simulink library "vmc"  (R2021b)
settings: Solver=VariableStepAuto  StartTime=0.0  StopTime=10.0  RelTol=1e-3
undefined symbols (not defined in the file): AVMC_ACCDeltaTqGradeGn_X_deg, AVMC_ACCDeltaTqIGain4OVRD_X_kph, AVMC_ACCDeltaTqIGain4OVRD_Y_mps2, AVMC_ACCDeltaTqIGain_X_kph, AVMC_ACCDeltaTqIGain_Y_mps2, AVMC_ACCDeltaTqPGain_X_kph, AVMC_ACCDeltaTqPGain_Y_kph, AVMC_ACCGradeofst_X_G, AVMC_ACCGradeofst_Y_pct, AVMC_ACCLoSpdTqLoLim4JP_X_kph, AVMC_ACCLoSpdTqLoLim4JP_Y_deg, AVMC_ACCLoSpdTqLowerLim_X_kph, AVMC_ACCLoSpdTqLowerLim_Y_deg, AVMC_ACCReqAccelGain_X_mps2, AVMC_ACCReqAccelGain_Y_enum, AVMC_ADSPosGFBDeltaTq_X_kph, AVMC_ADSPosGFBDeltaTq_Y_mps2, AVMC_AggressJerkPCT4AT_X_kph, AVMC_AggressJerkPCT_X_kph, AVMC_AggressLimitPCT4AT_X_kph, AVMC_AggressLimitPCT_X_kph, AVMC_DECGradeofst_X_G, AVMC_DECGradeofst_Y_pct, AVMC_DISCDeltaTqIGain_X_kph, AVMC_DISCDeltaTqIGain_Y_mps2, AVMC_DISCDeltaTqPGain_X_kph, AVMC_DISCDeltaTqPGain_Y_kph, AVMC_EPSForceSelect_X_enum, AVMC_EPSForceSelect_Y_enum, AVMC_EPSForceSelectD21_X_enum, AVMC_EPSForceSelectD21_Y_enum, AVMC_ESCRegenOut_X_kph, AVMC_ESCRegenOut_Y_Deg, AVMC_ESCRegenOutEnSpd_X_Deg, AVMC_EstPitchSlopeTs_X_kph, AVMC_GradeCompFlt_X_kph, AVMC_GyroYBandLo_X_Gps, AVMC_HoldResTq_X_kph, AVMC_ISOAccLimit_X_mps, AVMC_ISODecLimit_X_mps, AVMC_ISOJerk_X_mps, AVMC_LatESCRegenOut_X_kph, AVMC_LatESCRegenOut_Y_Deg, AVMC_LongAccDeadZone_X_kph, AVMC_LongAccFiltTsforP2_X_Gps, AVMC_MCPresBaseTq_X_bar, AVMC_MSAPedalOvrd_X_kph, AVMC_MSASpdBand_X_kph, AVMC_MSATqDownEndTq_X_kph, AVMC_MSATqDownTime_X_kph, AVMC_NegZCHoldTq_X_kph, AVMC_OPDDisSlideRate_X_Deg, AVMC_OVRD2ActSR2FCMCMD_X_mps2, AVMC_PedalTqRWhlRatio_X_Nm, AVMC_PedalTqRWhlRatio_Y_gps, AVMC_PedalTqRWhlSlipGain_X_rat, AVMC_PedalTqRWhlSlipGain_Y_kph, AVMC_PedalTqRWhSTRGGain_X_deg, AVMC_PedalTqRWhSTRGGain_Y_kph, AVMC_PosZCHoldTq_X_kph ... (+593)
libraries: hcu_lib x143, simulink x96, tqr x4, $bdroot x1, simulink_extras x1
(part 3 of 17)

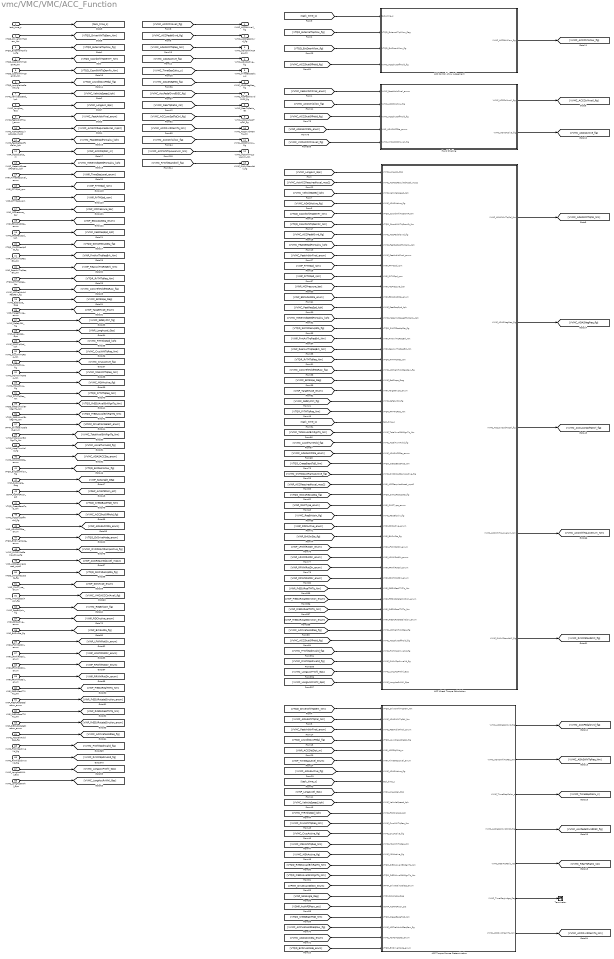
== system vmc/VMC/VMC/ACC_Function ==
  task_time_s : Inport
  VTQD_DriverWhlTqDem_Nm : Inport  Port=2
  VTQD_ExternalTqAllow_flg : Inport  Port=3
  VTQD_CoordWhlTqDemFr_Nm : Inport  Port=4
  VTQD_CoordWhlTqDemRr_Nm : Inport  Port=5
  VTQD_LowIdleAccPedal_flg : Inport  Port=6
  VVMC_VehicleSpeed_kph : Inport  Port=7
  VVMC_LongAcc_Gps : Inport  Port=8
  VVMC_FeatArbitrFinal_enum : Inport  Port=9
  VVMC_ActACCRequiredAccel_mps2 : Inport  Port=10
  VVMC_FeatSetSpdForCalcu_kph : Inport  Port=11
  VINP_ACCObjDist_m : Inport  Port=12
  VVMC_MeterIndSpeedForCalcu_kph : Inport  Port=13
  VINP_TimeGapLevel_enum : Inport  Port=14
  VINP_FrTMSpd_rpm : Inport  Port=15
  VINP_RrTMSpd_rpm : Inport  Port=16
  VINP_MCPressure_bar : Inport  Port=17
  VINP_ESCADASSta_enum : Inport  Port=18
  VVMC_FeatReqSpd_kph : Inport  Port=19
  VTQD_SWC2ResUpSta_flg : Inport  Port=20
  VINP_FrntAxlTrqReqBrk_Nm : Inport  Port=21
  VINP_RearAxlTrqReqBrk_Nm : Inport  Port=22
  VTQR_RrTMTqReq_Nm : Inport  Port=23
  VVMC_ACCVehHoldReqRaw_flg : Inport  Port=24
  VVMC_EstSlope_Deg : Inport  Port=25
  VINP_TargetType_enum : Inport  Port=26
  VVMC_SafetyCtrl_flg : Inport  Port=27
  VINP_LongAccel_Gps : Inport  Port=28
  VVMC_FrRrSlipSpd_kph : Inport  Port=29
  VVMC_CruzWhlTqReq_Nm : Inport  Port=30
  VVMC_CruzActive_flg : Inport  Port=31
  VVMC_MSAWhlTqReq_Nm : Inport  Port=32
  VVMC_MSAActive_flg : Inport  Port=33
  VTQR_FrTMTqReq_Nm : Inport  Port=34
  VTQD_RrEDUAvailBrkRgnTq_Nm : Inport  Port=35
  VTQD_FrEDUAvailBrkRgnTq_Nm : Inport  Port=36
  VPMM_DrivetrainSelect_enum : Inport  Port=37
  VVMC_TotalAvailBrkRgnTq_Nm : Inport  Port=38
  VVMC_AccelTurnHold_flg : Inport  Port=39
  VVMC_ADASACCSta_enum : Inport  Port=40
  VTQD_ExtDoorAllow_flg : Inport  Port=41
  VINP_SASAngle_Deg : Inport  Port=42
  VDHP_ActAPSPosn_pct : Inport  Port=43
  VTQD_CreepBaseTqD_Nm : Inport  Port=44
  VVMC_ACCShutOffHold_flg : Inport  Port=45
  VINP_ADASACCSta_enum : Inport  Port=46
  VTQD_EVDriveMode_enum : Inport  Port=47
  VVMC_OVRD2ActRampActive_flg : Inport  Port=48
  VINP_ACCRequiredAccel_mps2 : Inport  Port=49
  VTQD_SWC1ResUpSta_flg : Inport  Port=50
  VINP_SWCType_enum : Inport  Port=51
  VVMC_VMCACCCtrlAvail_flg : Inport  Port=52
  VVMC_ReqBrkJoin_flg : Inport  Port=53
  VINP_RDCActive_enum : Inport  Port=54
  VINP_BrkSwSta_flg : Inport  Port=55
  VINP_LFWhlRotDir_enum : Inport  Port=56
  VINP_LRWhlRotDir_enum : Inport  Port=57
  VINP_RFWhlRotDir_enum : Inport  Port=58
  VINP_RRWhlRotDir_enum : Inport  Port=59
  VINP_FrEDURealTMTq_Nm : Inport  Port=60
  VINP_FrEDURotateDirction_enum : Inport  Port=61
  VINP_RrEDURealTMTq_Nm : Inport  Port=62
  VINP_RrEDURotateDirction_enum : Inport  Port=63
  VVMC_ACCVehHoldReq_flg : Inport  Port=64
  VVMC_FrWhlSpdInvalid_flg : Inport  Port=65
  VVMC_RrWhlSpdInvalid_flg : Inport  Port=66
  VVMC_LongAccFrWhl_Gps : Inport  Port=67
  VVMC_LongAccRrWhl_Gps : Inport  Port=68
  ACC Control Allow Judgement : Subsystem
  ACC Torque Source Determination : Subsystem
  ACC Wheel Torque Calculation : Subsystem
  Hand Shaking : Subsystem
  Terminator : Terminator
  VVMC_ACCCtrlAvail_flg : Outport
  VVMC_ACCPedalOvrd_flg : Outport  Port=2
  VVMC_ADASWhlTqReq_Nm : Outport  Port=3
  VVMC_ADASActive_flg : Outport  Port=4
  VVMC_TimeGapCalcu_s : Outport  Port=5
  VVMC_ADASNegReq_flg : Outport  Port=6
  VVMC_AccPedalOvrdDISC_flg : Outport  Port=7
  VVMC_RearTqRatio_rat : Outport  Port=8
  VVMC_ACCLowSpdTqCtrl_flg : Outport  Port=9
  VVMC_ACCOvrdMemTq_Nm : Outport  Port=10
  VVMC_ACCCtrlAllow_flg : Outport  Port=11
  VVMC_ACCWhlTqLowerLim_Nm : Outport  Port=12
  VVMC_RrWhlStandstill_flg : Outport  Port=13
  wires:
  [VVMC_ACCCtrlAllow_flg] -> VVMC_ACCCtrlAllow_flg/1
  VVMC_VMCACCCtrlAvail_flg/1 -> [VVMC_VMCACCCtrlAvail_flg]
  [VVMC_VMCACCCtrlAvail_flg] -> Hand Shaking/5(VVMC_VMCACCCtrlAvail_flg)
  [VINP_SWCType_enum] -> ACC Wheel Torque Calculation/33(VINP_SWCType_enum)
  VINP_SWCType_enum/1 -> [VINP_SWCType_enum]
  [VTQD_SWC1ResUpSta_flg] -> ACC Wheel Torque Calculation/32(VTQD_SWC1ResUpSta_flg)
  VTQD_SWC1ResUpSta_flg/1 -> [VTQD_SWC1ResUpSta_flg]
  [VINP_ACCRequiredAccel_mps2] -> ACC Wheel Torque Calculation/31(VINP_ACCRequiredAccel_mps2)
  VINP_ACCRequiredAccel_mps2/1 -> [VINP_ACCRequiredAccel_mps2]
  [VVMC_OVRD2ActRampActive_flg] -> ACC Wheel Torque Calculation/30(VVMC_OVRD2ActRampActive_flg)
  VVMC_OVRD2ActRampActive_flg/1 -> [VVMC_OVRD2ActRampActive_flg]
  [VTQD_EVDriveMode_enum] -> ACC Torque Source Determination/24(VTQD_EVDriveMode_enum)
  VTQD_EVDriveMode_enum/1 -> [VTQD_EVDriveMode_enum]
  [VINP_ADASACCSta_enum] -> Hand Shaking/4(VINP_ADASACCSta_enum)
  VINP_ADASACCSta_enum/1 -> [VINP_ADASACCSta_enum]
  [VVMC_ACCShutOffHold_flg] -> Hand Shaking/3(VVMC_ACCShutOffHold_flg)
  VVMC_ACCShutOffHold_flg/1 -> [VVMC_ACCShutOffHold_flg]
  [VTQD_CreepBaseTqD_Nm] -> ACC Wheel Torque Calculation/29(VTQD_CreepBaseTqD_Nm)
  [VVMC_ADASACCSta_enum] -> ACC Torque Source Determination/23(VVMC_ADASACCSta_enum)
  [VVMC_ACCVehHoldReqRaw_flg] -> ACC Torque Source Determination/22(VVMC_ACCVehHoldReqRaw_flg)
  ACC Torque Source Determination/7(VVMC_ACCOvrdMemTq_Nm) -> [VVMC_ACCOvrdMemTq_Nm]
  [VVMC_ACCOvrdMemTq_Nm] -> VVMC_ACCOvrdMemTq_Nm/1
  [VTQD_CreepBaseTqD_Nm] -> ACC Torque Source Determination/21(VTQD_CreepBaseTqD_Nm)
  VTQD_CreepBaseTqD_Nm/1 -> [VTQD_CreepBaseTqD_Nm]
  VDHP_ActAPSPosn_pct/1 -> [VDHP_ActAPSPosn_pct]
  [VDHP_ActAPSPosn_pct] -> ACC Torque Source Determination/20(VDHP_ActAPSPosn_pct)
  VINP_SASAngle_Deg/1 -> [VINP_SASAngle_Deg]
  [VINP_SASAngle_Deg] -> ACC Torque Source Determination/19(VINP_SASAngle_Deg)
  VTQD_ExtDoorAllow_flg/1 -> [VTQD_ExtDoorAllow_flg]
  [VTQD_ExtDoorAllow_flg] -> ACC Control Allow Judgement/3(VTQD_ExtDoorAllow_flg)
  ACC Torque Source Determination/6(VVMC_TimeGapJudge_flag) -> Terminator/1
  [VVMC_ADASACCSta_enum] -> ACC Wheel Torque Calculation/28(VVMC_ADASACCSta_enum)
  VVMC_ADASACCSta_enum/1 -> [VVMC_ADASACCSta_enum]
  [VVMC_AccelTurnHold_flg] -> ACC Wheel Torque Calculation/27(VVMC_AccelTurnHold_flg)
  VVMC_AccelTurnHold_flg/1 -> [VVMC_AccelTurnHold_flg]
  [VVMC_TotalAvailBrkRgnTq_Nm] -> ACC Wheel Torque Calculation/26(VVMC_TotalAvailBrkRgnTq_Nm)
  VVMC_TotalAvailBrkRgnTq_Nm/1 -> [VVMC_TotalAvailBrkRgnTq_Nm]
  [task_time_s] -> ACC Wheel Torque Calculation/25(task_time_s)
  [VPMM_DrivetrainSelect_enum] -> ACC Torque Source Determination/18(VPMM_DrivetrainSelect_enum)
  VPMM_DrivetrainSelect_enum/1 -> [VPMM_DrivetrainSelect_enum]
  [VVMC_ACCLowSpdTqCtrl_flg] -> VVMC_ACCLowSpdTqCtrl_flg/1
  ACC Wheel Torque Calculation/3(VVMC_ACCLowSpdTqCtrl_flg) -> [VVMC_ACCLowSpdTqCtrl_flg]
  [VTQD_FrEDUAvailBrkRgnTq_Nm] -> ACC Torque Source Determination/17(VTQD_FrEDUAvailBrkRgnTq_Nm)
  [VTQD_RrEDUAvailBrkRgnTq_Nm] -> ACC Torque Source Determination/16(VTQD_RrEDUAvailBrkRgnTq_Nm)
  VTQD_FrEDUAvailBrkRgnTq_Nm/1 -> [VTQD_FrEDUAvailBrkRgnTq_Nm]
  VTQD_RrEDUAvailBrkRgnTq_Nm/1 -> [VTQD_RrEDUAvailBrkRgnTq_Nm]
  VTQR_FrTMTqReq_Nm/1 -> [VTQR_FrTMTqReq_Nm]
  [VTQR_FrTMTqReq_Nm] -> ACC Wheel Torque Calculation/24(VTQR_FrTMTqReq_Nm)
  [VVMC_MSAActive_flg] -> ACC Torque Source Determination/15(VVMC_MSAActive_flg)
  [VVMC_MSAWhlTqReq_Nm] -> ACC Torque Source Determination/14(VVMC_MSAWhlTqReq_Nm)
  [VVMC_CruzActive_flg] -> ACC Torque Source Determination/13(VVMC_CruzActive_flg)
  [VVMC_CruzWhlTqReq_Nm] -> ACC Torque Source Determination/12(VVMC_CruzWhlTqReq_Nm)
  VVMC_CruzWhlTqReq_Nm/1 -> [VVMC_CruzWhlTqReq_Nm]
  VVMC_CruzActive_flg/1 -> [VVMC_CruzActive_flg]
  VVMC_MSAWhlTqReq_Nm/1 -> [VVMC_MSAWhlTqReq_Nm]
  VVMC_MSAActive_flg/1 -> [VVMC_MSAActive_flg]
  [VVMC_FrRrSlipSpd_kph] -> ACC Torque Source Determination/11(VVMC_FrRrSlipSpd_kph)
  [VVMC_VehicleSpeed_kph] -> ACC Torque Source Determination/10(VVMC_VehicleSpeed_kph)
  VVMC_FrRrSlipSpd_kph/1 -> [VVMC_FrRrSlipSpd_kph]
  VINP_LongAccel_Gps/1 -> [VINP_LongAccel_Gps]
  [VVMC_RearTqRatio_rat] -> VVMC_RearTqRatio_rat/1
  ACC Torque Source Determination/5(VVMC_RearTqRatio_rat) -> [VVMC_RearTqRatio_rat]
  [VINP_LongAccel_Gps] -> ACC Torque Source Determination/9(VINP_LongAccel_Gps)
  [VVMC_SafetyCtrl_flg] -> ACC Wheel Torque Calculation/23(VVMC_SafetyCtrl_flg)
  VVMC_SafetyCtrl_flg/1 -> [VVMC_SafetyCtrl_flg]
  [task_time_s] -> ACC Torque Source Determination/8(task_time_s)
  VINP_TargetType_enum/1 -> [VINP_TargetType_enum]
  [VINP_TargetType_enum] -> ACC Wheel Torque Calculation/22(VINP_TargetType_enum)
  [VVMC_EstSlope_Deg] -> ACC Wheel Torque Calculation/21(VVMC_EstSlope_Deg)
  VVMC_EstSlope_Deg/1 -> [VVMC_EstSlope_Deg]
  [VVMC_ACCVehHoldReqRaw_flg] -> ACC Wheel Torque Calculation/20(VVMC_ACCVehHoldReqRaw_flg)
  VVMC_ACCVehHoldReqRaw_flg/1 -> [VVMC_ACCVehHoldReqRaw_flg]
  [VVMC_AccPedalOvrdDISC_flg] -> VVMC_AccPedalOvrdDISC_flg/1
  ACC Torque Source Determination/4(VVMC_AccPedalOvrdDISC_flg) -> [VVMC_AccPedalOvrdDISC_flg]
  [VTQR_RrTMTqReq_Nm] -> ACC Wheel Torque Calculation/19(VTQR_RrTMTqReq_Nm)
  VTQR_RrTMTqReq_Nm/1 -> [VTQR_RrTMTqReq_Nm]
  [VVMC_ADASNegReq_flg] -> VVMC_ADASNegReq_flg/1
  ACC Wheel Torque Calculation/2(VVMC_ADASNegReq_flg) -> [VVMC_ADASNegReq_flg]
  [VINP_RearAxlTrqReqBrk_Nm] -> ACC Wheel Torque Calculation/18(VINP_RearAxlTrqReqBrk_Nm)
  [VINP_FrntAxlTrqReqBrk_Nm] -> ACC Wheel Torque Calculation/17(VINP_FrntAxlTrqReqBrk_Nm)
  [VTQD_SWC2ResUpSta_flg] -> ACC Wheel Torque Calculation/16(VTQD_SWC2ResUpSta_flg)
  [VVMC_MeterIndSpeedForCalcu_kph] -> ACC Wheel Torque Calculation/15(VVMC_MeterIndSpeedForCalcu_kph)
  VINP_RearAxlTrqReqBrk_Nm/1 -> [VINP_RearAxlTrqReqBrk_Nm]
  VINP_FrntAxlTrqReqBrk_Nm/1 -> [VINP_FrntAxlTrqReqBrk_Nm]
  VTQD_SWC2ResUpSta_flg/1 -> [VTQD_SWC2ResUpSta_flg]
  [VVMC_FeatSetSpdForCalcu_kph] -> ACC Wheel Torque Calculation/8(VVMC_FeatSetSpdForCalcu_kph)
  VVMC_FeatSetSpdForCalcu_kph/1 -> [VVMC_FeatSetSpdForCalcu_kph]
  [VTQD_LowIdleAccPedal_flg] -> ACC Torque Source Determination/4(VTQD_LowIdleAccPedal_flg)
  VTQD_LowIdleAccPedal_flg/1 -> [VTQD_LowIdleAccPedal_flg]
  [VVMC_FeatArbitrFinal_enum] -> ACC Torque Source Determination/3(VVMC_FeatArbitrFinal_enum)
  [VVMC_ACCPedalOvrd_flg] -> ACC Wheel Torque Calculation/7(VVMC_ACCPedalOvrd_flg)
  VTQD_CoordWhlTqDemFr_Nm/1 -> [VTQD_CoordWhlTqDemFr_Nm]
  VTQD_CoordWhlTqDemRr_Nm/1 -> [VTQD_CoordWhlTqDemRr_Nm]
  [VTQD_CoordWhlTqDemRr_Nm] -> ACC Wheel Torque Calculation/6(VTQD_CoordWhlTqDemRr_Nm)
  [VTQD_CoordWhlTqDemFr_Nm] -> ACC Wheel Torque Calculation/5(VTQD_CoordWhlTqDemFr_Nm)
  [VVMC_ADASWhlTqReq_Nm] -> VVMC_ADASWhlTqReq_Nm/1
  ACC Torque Source Determination/2(VVMC_ADASWhlTqReq_Nm) -> [VVMC_ADASWhlTqReq_Nm]
  [VVMC_ADASActive_flg] -> VVMC_ADASActive_flg/1
  [VVMC_ACCCtrlAllow_flg] -> Hand Shaking/2(VVMC_ACCCtrlAllow_flg)
  task_time_s/1 -> [task_time_s]
  [VVMC_ADASActive_flg] -> ACC Wheel Torque Calculation/4(VVMC_ADASActive_flg)
  Hand Shaking/2(VVMC_ADASActive_flg) -> [VVMC_ADASActive_flg]
  [VVMC_FeatArbitrFinal_enum] -> Hand Shaking/1(VVMC_FeatArbitrFinal_enum)
  ACC Torque Source Determination/1(VVMC_ACCPedalOvrd_flg) -> [VVMC_ACCPedalOvrd_flg]
  [VVMC_ADASWhlTqCal_Nm] -> ACC Torque Source Determination/2(VVMC_ADASWhlTqCal_Nm)
  [VTQD_DriverWhlTqDem_Nm] -> ACC Torque Source Determination/1(VTQD_DriverWhlTqDem_Nm)
  ACC Wheel Torque Calculation/1(VVMC_ADASWhlTqCal_Nm) -> [VVMC_ADASWhlTqCal_Nm]
  [VVMC_VehicleSpeed_kph] -> ACC Wheel Torque Calculation/3(VVMC_VehicleSpeed_kph)
  [VVMC_ActACCRequiredAccel_mps2] -> ACC Wheel Torque Calculation/2(VVMC_ActACCRequiredAccel_mps2)
  [VVMC_LongAcc_Gps] -> ACC Wheel Torque Calculation/1(VVMC_LongAcc_Gps)
  VTQD_DriverWhlTqDem_Nm/1 -> [VTQD_DriverWhlTqDem_Nm]
  VVMC_VehicleSpeed_kph/1 -> [VVMC_VehicleSpeed_kph]
  VTQD_ExternalTqAllow_flg/1 -> [VTQD_ExternalTqAllow_flg]
  [VVMC_ACCCtrlAvail_flg] -> VVMC_ACCCtrlAvail_flg/1
  VVMC_ActACCRequiredAccel_mps2/1 -> [VVMC_ActACCRequiredAccel_mps2]
  VVMC_FeatArbitrFinal_enum/1 -> [VVMC_FeatArbitrFinal_enum]
  VVMC_LongAcc_Gps/1 -> [VVMC_LongAcc_Gps]
  Hand Shaking/1(VVMC_ACCCtrlAvail_flg) -> [VVMC_ACCCtrlAvail_flg]
  [VVMC_ACCPedalOvrd_flg] -> VVMC_ACCPedalOvrd_flg/1
  VVMC_MeterIndSpeedForCalcu_kph/1 -> [VVMC_MeterIndSpeedForCalcu_kph]
  VINP_ACCObjDist_m/1 -> [VINP_ACCObjDist_m]
  VINP_TimeGapLevel_enum/1 -> [VINP_TimeGapLevel_enum]
  [VINP_ACCObjDist_m] -> ACC Torque Source Determination/5(VINP_ACCObjDist_m)
  [VINP_TimeGapLevel_enum] -> ACC Torque Source Determination/6(VINP_TimeGapLevel_enum)
  ACC Torque Source Determination/3(VVMC_TimeGapCalcu_s) -> [VVMC_TimeGapCalcu_s]
  [VVMC_TimeGapCalcu_s] -> VVMC_TimeGapCalcu_s/1
  [task_time_s] -> ACC Control Allow Judgement/1(task_time_s)
  ACC Control Allow Judgement/1(VVMC_ACCCtrlAllow_flg) -> [VVMC_ACCCtrlAllow_flg]
  [VTQD_ExternalTqAllow_flg] -> ACC Control Allow Judgement/2(VTQD_ExternalTqAllow_flag)
  [VVMC_FeatArbitrFinal_enum] -> ACC Wheel Torque Calculation/9(VVMC_FeatArbitrFinal_enum)
  VINP_ESCADASSta_enum/1 -> [VINP_ESCADASSta_enum]
  VINP_MCPressure_bar/1 -> [VINP_MCPressure_bar]
  VINP_RrTMSpd_rpm/1 -> [VINP_RrTMSpd_rpm]
  VINP_FrTMSpd_rpm/1 -> [VINP_FrTMSpd_rpm]
  [VINP_FrTMSpd_rpm] -> ACC Wheel Torque Calculation/10(VINP_FrTMSpd_rpm)
  [VINP_RrTMSpd_rpm] -> ACC Wheel Torque Calculation/11(VINP_RrTMSpd_rpm)
  [VINP_MCPressure_bar] -> ACC Wheel Torque Calculation/12(VINP_MCPressure_bar)
  [VINP_ESCADASSta_enum] -> ACC Wheel Torque Calculation/13(VINP_ESCADASSta_enum)
  [VVMC_ADASActive_flg] -> ACC Torque Source Determination/7(VVMC_ADASActive_flg)
  VVMC_FeatReqSpd_kph/1 -> [VVMC_FeatReqSpd_kph]
  [VVMC_FeatReqSpd_kph] -> ACC Wheel Torque Calculation/14(VVMC_FeatReqSpd_kph)
  VVMC_ReqBrkJoin_flg/1 -> [VVMC_ReqBrkJoin_flg]
  [VVMC_ReqBrkJoin_flg] -> ACC Wheel Torque Calculation/34(VVMC_ReqBrkJoin_flg)
  [VVMC_ACCWhlTqLowerLim_Nm] -> VVMC_ACCWhlTqLowerLim_Nm/1
  ACC Wheel Torque Calculation/4(VVMC_ACCWhlTqLowerLim_Nm) -> [VVMC_ACCWhlTqLowerLim_Nm]
  VINP_RDCActive_enum/1 -> [VINP_RDCActive_enum]
  [VINP_RDCActive_enum] -> ACC Wheel Torque Calculation/35(VINP_RDCActive_enum)
  VINP_BrkSwSta_flg/1 -> [VINP_BrkSwSta_flg]
  [VINP_BrkSwSta_flg] -> ACC Wheel Torque Calculation/36(VINP_BrkSwSta_flg)
  VINP_LFWhlRotDir_enum/1 -> [VINP_LFWhlRotDir_enum]
  VINP_RFWhlRotDir_enum/1 -> [VINP_RFWhlRotDir_enum]
  VINP_LRWhlRotDir_enum/1 -> [VINP_LRWhlRotDir_enum]
  VINP_RRWhlRotDir_enum/1 -> [VINP_RRWhlRotDir_enum]
  [VINP_LFWhlRotDir_enum] -> ACC Wheel Torque Calculation/37(VINP_LFWhlRotDir_enum)
  [VINP_LRWhlRotDir_enum] -> ACC Wheel Torque Calculation/38(VINP_LRWhlRotDir_enum)
  [VINP_RFWhlRotDir_enum] -> ACC Wheel Torque Calculation/39(VINP_RFWhlRotDir_enum)
  [VINP_RRWhlRotDir_enum] -> ACC Wheel Torque Calculation/40(VINP_RRWhlRotDir_enum)
  VINP_FrEDURotateDirction_enum/1 -> [VINP_FrEDURotateDirction_enum]
  VINP_RrEDURotateDirction_enum/1 -> [VINP_RrEDURotateDirction_enum]
  VINP_FrEDURealTMTq_Nm/1 -> [VINP_FrEDURealTMTq_Nm]
  VINP_RrEDURealTMTq_Nm/1 -> [VINP_RrEDURealTMTq_Nm]
  [VINP_FrEDURealTMTq_Nm] -> ACC Wheel Torque Calculation/41(VINP_FrEDURealTMTq_Nm)
  [VINP_FrEDURotateDirction_enum] -> ACC Wheel Torque Calculation/42(VINP_FrEDURotateDirction_enum)
  [VINP_RrEDURealTMTq_Nm] -> ACC Wheel Torque Calculation/43(VINP_RrEDURealTMTq_Nm)
  [VINP_RrEDURotateDirction_enum] -> ACC Wheel Torque Calculation/44(VINP_RrEDURotateDirction_enum)
  [VVMC_RrWhlStandstill_flg] -> VVMC_RrWhlStandstill_flg/1
  ACC Wheel Torque Calculation/5(VVMC_RrWhlStandstill_flg) -> [VVMC_RrWhlStandstill_flg]
  [VVMC_ACCShutOffHold_flg] -> ACC Control Allow Judgement/4(VVMC_ACCShutOffHold_flg)
  VVMC_ACCVehHoldReq_flg/1 -> [VVMC_ACCVehHoldReq_flg]
  [VVMC_ACCVehHoldReq_flg] -> ACC Wheel Torque Calculation/45(VVMC_ACCVehHoldReq_flg)
  [VVMC_ACCShutOffHold_flg] -> ACC Wheel Torque Calculation/46(VVMC_ACCShutOffHold_flg)
  VVMC_FrWhlSpdInvalid_flg/1 -> [VVMC_FrWhlSpdInvalid_flg]
  VVMC_RrWhlSpdInvalid_flg/1 -> [VVMC_RrWhlSpdInvalid_flg]
  VVMC_LongAccFrWhl_Gps/1 -> [VVMC_LongAccFrWhl_Gps]
  VVMC_LongAccRrWhl_Gps/1 -> [VVMC_LongAccRrWhl_Gps]
  [VVMC_FrWhlSpdInvalid_flg] -> ACC Wheel Torque Calculation/47(VVMC_FrWhlSpdInvalid_flg)
  [VVMC_RrWhlSpdInvalid_flg] -> ACC Wheel Torque Calculation/48(VVMC_RrWhlSpdInvalid_flg)
  [VVMC_LongAccFrWhl_Gps] -> ACC Wheel Torque Calculation/49(VVMC_LongAccFrWhl_Gps)
  [VVMC_LongAccRrWhl_Gps] -> ACC Wheel Torque Calculation/50(VVMC_LongAccRrWhl_Gps)

== system vmc/VMC/VMC/APS function ==
  VTQD_ExternalTqAllow_flg : Inport
  VTQD_ExtShiftAllow_flg : Inport  Port=2
  VTQD_ExtDoorAllow_flg : Inport  Port=3
  VTQD_GearActualPosn_enum : Inport  Port=4
  VINP_APSVMCReqA_flg : Inport  Port=5
  VINP_APSShiftPosnReq_enum : Inport  Port=6
  VINP_APSSpeedCMD_kph : Inport  Port=7
  task_time_s : Inport  Port=8
  VINP_SCPSystemMode_enum : Inport  Port=9
  VVMC_ADASActive_flg : Inport  Port=10
  VTQD_APSStaSys_enum : Inport  Port=11
  VTQD_APSDecReqA_flg : Inport  Port=12
  VTQD_APSDecReq_mps2 : Inport  Port=13
  VTQD_APSReq_enum : Inport  Port=14
  VINP_APSStaSystem_enum : Inport  Port=15
  VINP_APSDecReqA_flg : Inport  Port=16
  VINP_APSDecReq_mps2 : Inport  Port=17
  VINP_APSReq_enum : Inport  Port=18
  VVMC_VehicleSpeed_kph : Inport  Port=19
  VVMC_CruzActive_flg : Inport  Port=20
  VINP_CAASVMCReqA_flg : Inport  Port=21
  VINP_ADASACCSta_enum : Inport  Port=22
  VINP_BrkSwSta_flg : Inport  Port=23
  VINP_MCPressure_bar : Inport  Port=24
  VINP_BrkPedalPos_pct : Inport  Port=25
  VINP_ACCObjDist_m : Inport  Port=26
  VVMC_MeterIndSpeedForCalcu_kph : Inport  Port=27
  VDDM_VCURAPSErrLv2_flg : Inport  Port=28
  VDDM_VCURAPSErrLv3_flg : Inport  Port=29
  VTQD_EPBCarWashMode_flg : Inport  Port=30
  CAAS HandShake : Subsystem
  Command Determination1 : Subsystem
  Hand Shake : Subsystem
  Signal Rounting : Subsystem
  Subsystem : Subsystem
  VVMC_APSCtrlAvail_flg : Outport
  VVMC_APSActive_flg : Outport  Port=2
  VVMC_CAASCtrlAvail_flg : Outport  Port=3
  VVMC_CAASActive_flg : Outport  Port=4
  VVMC_APSSpeedCMD_kph : Outport  Port=5
  VVMC_APSShiftPosnReq_enum : Outport  Port=6
  VVMC_APSStaSys_enum : Outport  Port=7
  VVMC_APSDecReqA_flg : Outport  Port=8
  VVMC_APSDecReq_mps2 : Outport  Port=9
  VVMC_APSReq_enum : Outport  Port=10
  VVMC_SetACCDisableAPS_flg : Outport  Port=11
  wires:
  VDDM_VCURAPSErrLv2_flg/1 -> [VDDM_VCURAPSErrLv2_flg]
  VTQD_EPBCarWashMode_flg/1 -> [VTQD_EPBCarWashMode_flg]
  VDDM_VCURAPSErrLv3_flg/1 -> [VDDM_VCURAPSErrLv3_flg]
  [VTQD_EPBCarWashMode_flg] -> Hand Shake/10(VTQD_EPBCarWashMode_flg)
  [VTQD_GearActualPosn_enum] -> Hand Shake/7(VTQD_GearActualPosn_enum)
  [VDDM_VCURAPSErrLv2_flg] -> Hand Shake/8(VDDM_VCURAPSErrLv2_flg)
  [VDDM_VCURAPSErrLv3_flg] -> Hand Shake/9(VDDM_VCURAPSErrLv3_flg)
  [VVMC_VehicleSpeed_kph] -> Subsystem/8(VVMC_VehicleSpeed_kph)
  [VVMC_SetACCDisableAPS_flg] -> Signal Rounting/14(VVMC_SetACCDisableAPS_flg)
  VVMC_MeterIndSpeedForCalcu_kph/1 -> [VVMC_MeterIndSpeedForCalcu_kph]
  VINP_ACCObjDist_m/1 -> [VINP_ACCObjDist_m]
  VINP_BrkPedalPos_pct/1 -> [VINP_BrkPedalPos_pct]
  VINP_MCPressure_bar/1 -> [VINP_MCPressure_bar]
  VINP_BrkSwSta_flg/1 -> [VINP_BrkSwSta_flg]
  VINP_ADASACCSta_enum/1 -> [VINP_ADASACCSta_enum]
  Subsystem/1(VVMC_SetACCDisableAPS_flg) -> [VVMC_SetACCDisableAPS_flg], VVMC_SetACCDisableAPS_flg/1
  [VINP_ADASACCSta_enum] -> Subsystem/1(VINP_ADASACCSta_enum)
  [VVMC_MeterIndSpeedForCalcu_kph] -> Subsystem/7(VVMC_MeterIndSpeedForCalcu_kph)
  [VINP_ACCObjDist_m] -> Subsystem/6(VINP_ACCObjDist_m)
  [VINP_BrkSwSta_flg] -> Subsystem/3(VINP_BrkSwSta_flg)
  [VINP_MCPressure_bar] -> Subsystem/2(VINP_MCPressure_bar)
  [VINP_BrkPedalPos_pct] -> Subsystem/4(VINP_BrkPedalPos_pct)
  [VTQD_APSDecReqA_flg] -> Subsystem/5(VTQD_APSDecReqA_flg)
  VINP_CAASVMCReqA_flg/1 -> [VINP_CAASVMCReqA_flg]
  VVMC_CruzActive_flg/1 -> [VVMC_CruzActive_flg]
  VVMC_VehicleSpeed_kph/1 -> [VVMC_VehicleSpeed_kph]
  [VTQD_APSReq_enum] -> Signal Rounting/9(VTQD_APSReq_enum)
  [VINP_APSReq_enum] -> Signal Rounting/13(VINP_APSReq_enum)
  [VINP_APSDecReq_mps2] -> Signal Rounting/12(VINP_APSDecReq_mps2)
  [VINP_APSDecReqA_flg] -> Signal Rounting/11(VINP_APSDecReqA_flg)
  [VTQD_APSDecReq_mps2] -> Signal Rounting/8(VTQD_APSDecReq_mps2)
  [VTQD_APSDecReqA_flg] -> Signal Rounting/7(VTQD_APSDecReqA_flg)
  [VINP_APSStaSystem_enum] -> Signal Rounting/10(VINP_APSStaSystem_enum)
  [VTQD_APSStaSys_enum] -> Signal Rounting/6(VTQD_APSStaSys_enum)
  VINP_APSDecReqA_flg/1 -> [VINP_APSDecReqA_flg]
  VINP_APSStaSystem_enum/1 -> [VINP_APSStaSystem_enum]
  VINP_APSReq_enum/1 -> [VINP_APSReq_enum]
  VINP_APSDecReq_mps2/1 -> [VINP_APSDecReq_mps2]
  Signal Rounting/4(VVMC_APSReq_enum) -> VVMC_APSReq_enum/1
  [VINP_APSSpeedCMD_kph] -> Command Determination1/4(VINP_APSSpeedCMD_kph)
  Command Determination1/2(VVMC_APSShiftPosnReq_enum) -> VVMC_APSShiftPosnReq_enum/1
  [VINP_APSShiftPosnReq_enum] -> Command Determination1/3(VINP_APSShiftPosnReq_enum)
  [VINP_APSStaSystem_enum] -> Command Determination1/2(VINP_APSStaSys_enum)
  [VTQD_GearActualPosn_enum] -> Signal Rounting/4(VTQD_GearActualPosn_enum)
  [VINP_SCPSystemMode_enum] -> Signal Rounting/1(VINP_SCPSystemMode_enum)
  [VVMC_APSActive_flg] -> Signal Rounting/2(VVMC_APSActive_flg)
  Signal Rounting/1(VVMC_APSStaSys_enum) -> VVMC_APSStaSys_enum/1
  [VVMC_ADASActive_flg] -> Signal Rounting/3(VVMC_ADASActive_flg)
  Signal Rounting/3(VVMC_APSDecReq_mps2) -> VVMC_APSDecReq_mps2/1
  Signal Rounting/2(VVMC_APSDecReqA_flg) -> VVMC_APSDecReqA_flg/1
  [VVMC_APSActive_flg] -> Command Determination1/1(VVMC_APSActive_flg)
  [VVMC_CAASActive_flg] -> Signal Rounting/5(VVMC_CAASActive_flg)
  Command Determination1/1(VVMC_APSSpeedCMD_kph) -> VVMC_APSSpeedCMD_kph/1
  [VTQD_ExternalTqAllow_flg] -> Hand Shake/2(VTQD_ExternalTqAllow_flg)
  [task_time_s] -> Hand Shake/1(task_time_s)
  [VTQD_ExtShiftAllow_flg] -> Hand Shake/3(VTQD_ExtShiftAllow_flg)
  [VINP_APSStaSystem_enum] -> Hand Shake/5(VINP_APSStaSys_enum)
  CAAS HandShake/2(VVMC_CAASActive_flg) -> [VVMC_CAASActive_flg], VVMC_CAASActive_flg/1
  [VINP_CAASVMCReqA_flg] -> CAAS HandShake/5(VINP_CAASVMCReqA_flg)
  [task_time_s] -> CAAS HandShake/4(task_time_s)
  CAAS HandShake/1(VVMC_CAASCtrlAvail_flg) -> VVMC_CAASCtrlAvail_flg/1
  [VINP_APSVMCReqA_flg] -> Hand Shake/4(VINP_APSVMCReqA_flg)
  [VVMC_ADASActive_flg] -> CAAS HandShake/2(VVMC_ADASActive_flg)
  [VVMC_VehicleSpeed_kph] -> CAAS HandShake/1(VVMC_VehicleSpeed_kph)
  [VVMC_CruzActive_flg] -> CAAS HandShake/3(VVMC_CruzActive_flg)
  Hand Shake/2(VVMC_APSActive_flg) -> [VVMC_APSActive_flg], VVMC_APSActive_flg/1
  [VTQD_ExtDoorAllow_flg] -> Hand Shake/6(VTQD_ExtDoorAllow_flg)
  Hand Shake/1(VVMC_APSCtrlAvail_flg) -> VVMC_APSCtrlAvail_flg/1
  VTQD_APSReq_enum/1 -> [VTQD_APSReq_enum]
  VTQD_APSDecReqA_flg/1 -> [VTQD_APSDecReqA_flg]
  VTQD_APSDecReq_mps2/1 -> [VTQD_APSDecReq_mps2]
  VTQD_APSStaSys_enum/1 -> [VTQD_APSStaSys_enum]
  VINP_SCPSystemMode_enum/1 -> [VINP_SCPSystemMode_enum]
  VTQD_GearActualPosn_enum/1 -> [VTQD_GearActualPosn_enum]
  VTQD_ExtShiftAllow_flg/1 -> [VTQD_ExtShiftAllow_flg]
  VTQD_ExternalTqAllow_flg/1 -> [VTQD_ExternalTqAllow_flg]
  VTQD_ExtDoorAllow_flg/1 -> [VTQD_ExtDoorAllow_flg]
  VVMC_ADASActive_flg/1 -> [VVMC_ADASActive_flg]
  VINP_APSVMCReqA_flg/1 -> [VINP_APSVMCReqA_flg]
  VINP_APSShiftPosnReq_enum/1 -> [VINP_APSShiftPosnReq_enum]
  VINP_APSSpeedCMD_kph/1 -> [VINP_APSSpeedCMD_kph]
  task_time_s/1 -> [task_time_s]

== system vmc/VMC/VMC/CruiseControlFunction ==
  VTQD_ExternalTqAllow_flg : Inport
  VTQD_DriverWhlTqDem_Nm : Inport  Port=2
  VTQD_LowIdleAccPedal_flg : Inport  Port=3
  <VTQD_SpdCtrlMode_enum> : Inport  Port=4
  VTQD_SWC1ResUpSta_flg : Inport  Port=5
  VTQD_SWC1SetdownSta_flg : Inport  Port=6
  VTQD_SWC1CANCELSta_flg : Inport  Port=7
  VINP_BrakeSWGPIO_flg : Inport  Port=8
  VINP_BrkSwSta_flg : Inport  Port=9
  VVMC_VehicleSpeed_kph : Inport  Port=10
  VVMC_LongAcc_Gps : Inport  Port=11
  VVMC_FeatSetSpdForCalcu_kph : Inport  Port=12
  VVMC_FeatArbitrFinal_enum : Inport  Port=13
  VINP_ADASAEBSta_enum : Inport  Port=14
  VTQD_GearActualPosn_enum : Inport  Port=15
  VVMC_SafetyCtrl_flg : Inport  Port=16
  VTQR_FrTMTqReq_Nm : Inport  Port=17
  VTQR_RrTMTqReq_Nm : Inport  Port=18
  VTQD_RegenMode_enum : Inport  Port=19
  VVMC_ActACCRequiredAccel_mps2 : Inport  Port=20
  task_time_s : Inport  Port=21
  VVMC_TotalAvailBrkRgnTq_Nm : Inport  Port=22
  VINP_Distanceunit_flg : Inport  Port=23
  VTQD_ExtDoorAllow_flg : Inport  Port=24
  VVMC_VMCCCCtrlAvail_flg : Inport  Port=25
  VVMC_FeatSetSpdFinal_raw32 : Inport  Port=26
  VVMC_MeterIndSpeed_raw32 : Inport  Port=27
  VINP_RDCActive_enum : Inport  Port=28
  CCActiveDetermination : Subsystem
  CCDemandTorqueCalculation : Subsystem
  CCTorqueSourceDetermination : Subsystem
  Data Type Conversion : DataTypeConversion  OutDataTypeStr=single
  VVMC_CCCtrlSta_enum : Outport
  VVMC_CCSpdWar_flg : Outport  Port=2
  VVMC_CruzWhlTqReq_Nm : Outport  Port=3
  VVMC_CruzActive_flg : Outport  Port=4
  VVMC_CCPedalOvrd_flg : Outport  Port=5
  wires:
  VVMC_FeatSetSpdFinal_raw32/1 -> [VVMC_FeatSetSpdFinal_raw32]
  [VVMC_VMCCCCtrlAvail_flg] -> CCActiveDetermination/16(VVMC_VMCCCCtrlAvail_flg)
  VVMC_VMCCCCtrlAvail_flg/1 -> [VVMC_VMCCCCtrlAvail_flg]
  [VTQD_ExtDoorAllow_flg] -> CCActiveDetermination/15(VTQD_ExtDoorAllow_flg)
  VTQD_ExtDoorAllow_flg/1 -> [VTQD_ExtDoorAllow_flg]
  VINP_Distanceunit_flg/1 -> [VINP_Distanceunit_flg]
  [VINP_Distanceunit_flg] -> CCActiveDetermination/14(VINP_Distanceunit_flg)
  [VVMC_TotalAvailBrkRgnTq_Nm] -> CCDemandTorqueCalculation/10(VVMC_TotalAvailBrkRgnTq_Nm)
  VVMC_TotalAvailBrkRgnTq_Nm/1 -> [VVMC_TotalAvailBrkRgnTq_Nm]
  [VVMC_ActACCRequiredAccel_mps2] -> CCDemandTorqueCalculation/6(VVMC_ActACCRequiredAccel_mps2)
  task_time_s/1 -> [task_time_s]
  VVMC_ActACCRequiredAccel_mps2/1 -> [VVMC_ActACCRequiredAccel_mps2]
  [task_time_s] -> CCTorqueSourceDetermination/6(task_time_s)
  VTQD_RegenMode_enum/1 -> [VTQD_RegenMode_enum]
  [VVMC_FeatArbitrFinal_enum] -> CCTorqueSourceDetermination/5(VVMC_FeatArbitrFinal_enum)
  [VTQD_RegenMode_enum] -> CCTorqueSourceDetermination/4(VTQD_RegenMode_enum)
  VTQR_RrTMTqReq_Nm/1 -> [VTQR_RrTMTqReq_Nm]
  VTQR_FrTMTqReq_Nm/1 -> [VTQR_FrTMTqReq_Nm]
  [VTQR_RrTMTqReq_Nm] -> CCDemandTorqueCalculation/9(VTQR_RrTMTqReq_Nm)
  [VTQR_FrTMTqReq_Nm] -> CCDemandTorqueCalculation/8(VTQR_FrTMTqReq_Nm)
  VVMC_SafetyCtrl_flg/1 -> [VVMC_SafetyCtrl_flg]
  [VVMC_SafetyCtrl_flg] -> CCDemandTorqueCalculation/7(VVMC_SafetyCtrl_flg)
  [VTQD_GearActualPosn_enum] -> CCActiveDetermination/13(VTQD_GearActualPosn_enum)
  VTQD_GearActualPosn_enum/1 -> [VTQD_GearActualPosn_enum]
  [VVMC_CCPedalOvrd_flg] -> CCDemandTorqueCalculation/5(VVMC_CCPedalOvrd_flg)
  CCTorqueSourceDetermination/2(VVMC_CCPedalOvrd_flg) -> [VVMC_CCPedalOvrd_flg]  "VVMC_CCPedalOvrd_flg"
  [VTQD_LowIdleAccPedal_flg] -> CCTorqueSourceDetermination/3(VTQD_LowIdleAccPedal_flg)
  VTQD_LowIdleAccPedal_flg/1 -> [VTQD_LowIdleAccPedal_flg]
  [VVMC_VehicleSpeed_kph] -> CCActiveDetermination/6(VVMC_VehicleSpeed_kph)
  [VVMC_LongAcc_Gps] -> CCDemandTorqueCalculation/4(VVMC_LongAcc_Gps)
  VVMC_LongAcc_Gps/1 -> [VVMC_LongAcc_Gps]
  [VVMC_CruzActive_flg] -> VVMC_CruzActive_flg/1
  Data Type Conversion/1 -> [VVMC_FeatSetSpdForCalcu_kph]  "VVMC_FeatSetSpdForCalcu_kph"
  [VVMC_CruzWhlTqReq_Nm] -> VVMC_CruzWhlTqReq_Nm/1
  [VVMC_CCSpdWar_flg] -> VVMC_CCSpdWar_flg/1
  [VVMC_CCCtrlSta_enum] -> VVMC_CCCtrlSta_enum/1
  VVMC_VehicleSpeed_kph/1 -> [VVMC_VehicleSpeed_kph]
  VVMC_FeatArbitrFinal_enum/1 -> [VVMC_FeatArbitrFinal_enum]
  VINP_BrkSwSta_flg/1 -> [VINP_BrkSwSta_flg]
  VVMC_FeatSetSpdForCalcu_kph/1 -> Data Type Conversion/1
  VINP_BrakeSWGPIO_flg/1 -> [VINP_BrakeSWGPIO_flg]
  VTQD_SWC1CANCELSta_flg/1 -> [VTQD_SWC1CANCELSta_flg]
  VTQD_SWC1SetdownSta_flg/1 -> [VTQD_SWC1SetdownSta_flg]
  VTQD_SWC1ResUpSta_flg/1 -> [VTQD_SWC1ResUpSta_flg]
  VTQD_DriverWhlTqDem_Nm/1 -> [VTQD_DriverWhlTqDem_Nm]
  VTQD_ExternalTqAllow_flg/1 -> [VTQD_ExternalTqAllow_flg]
  CCTorqueSourceDetermination/1(VVMC_CruzWhlTqReq_Nm) -> [VVMC_CruzWhlTqReq_Nm]  "VVMC_CruzWhlTqReq_Nm"
  CCDemandTorqueCalculation/1(VVMC_CruzWhlTqCal_Nm) -> [VVMC_CruzWhlTqCal_Nm]
  CCActiveDetermination/3(VVMC_CruzActive_flg) -> [VVMC_CruzActive_flg]
  CCActiveDetermination/2(VVMC_CCSpdWar_flg) -> [VVMC_CCSpdWar_flg]
  CCActiveDetermination/1(VVMC_CCCtrlSta_enum) -> [VVMC_CCCtrlSta_enum]
  [VVMC_CruzWhlTqCal_Nm] -> CCTorqueSourceDetermination/2(VVMC_CruzWhlTqCal_Nm)
  [VTQD_DriverWhlTqDem_Nm] -> CCTorqueSourceDetermination/1(VTQD_DriverWhlTqDem_Nm)
  [VVMC_CruzActive_flg] -> CCDemandTorqueCalculation/3(VVMC_CruzActive_flg)
  [VVMC_VehicleSpeed_kph] -> CCDemandTorqueCalculation/2(VVMC_VehicleSpeed_kph)
  [VVMC_FeatSetSpdForCalcu_kph] -> CCDemandTorqueCalculation/1(VVMC_FeatSetSpdForCalcu_kph)
  [VINP_BrkSwSta_flg] -> CCActiveDetermination/10(VINP_BrkSwSta_flg)
  [VTQD_SWC1CANCELSta_flg] -> CCActiveDetermination/9(VTQD_SWC1CANCELSta_flg)
  [VINP_BrakeSWGPIO_flg] -> CCActiveDetermination/8(VINP_BrakeSWGPIO_flg)
  [VVMC_FeatSetSpdFinal_raw32] -> CCActiveDetermination/7(VVMC_FeatSetSpdFinal_raw32)
  [VTQD_SWC1ResUpSta_flg] -> CCActiveDetermination/5(VTQD_SWC1ResUpSta_flg)
  [VTQD_SWC1SetdownSta_flg] -> CCActiveDetermination/4(VTQD_SWC1SetdownSta_flg)
  [VTQD_ExternalTqAllow_flg] -> CCActiveDetermination/3(VTQD_ExternalTqAllow_flg)
  [VVMC_FeatArbitrFinal_enum] -> CCActiveDetermination/2(VVMC_FeatArbitrFinal_enum)
  <VTQD_SpdCtrlMode_enum>/1 -> [VTQD_SpdCtrlMode_enum]
  [VTQD_SpdCtrlMode_enum] -> CCActiveDetermination/1(VTQD_SpdCtrlMode_enum)
  VINP_ADASAEBSta_enum/1 -> [VINP_ADASAEBSta_enum]
  [VINP_ADASAEBSta_enum] -> CCActiveDetermination/11(VINP_ADASAEBSta_enum)
  [VVMC_CCPedalOvrd_flg] -> CCActiveDetermination/12(VVMC_CCPedalOvrd_flg)
  [VVMC_CCPedalOvrd_flg] -> VVMC_CCPedalOvrd_flg/1
  VVMC_MeterIndSpeed_raw32/1 -> [VVMC_MeterIndSpeed_raw32]
  [VVMC_MeterIndSpeed_raw32] -> CCActiveDetermination/17(VVMC_MeterIndSpeed_raw32)
  VINP_RDCActive_enum/1 -> [VINP_RDCActive_enum]
  [VINP_RDCActive_enum] -> CCDemandTorqueCalculation/11(VINP_RDCActive_enum)

== system vmc/VMC/VMC/EPSForceSelect ==
  VINP_IVIEPSForceCmd_enum : Inport
  VPMM_DrivetrainSelect_enum : Inport  Port=2
  VINP_VehicleType_enum : Inport  Port=3
  Cast To Single : DataTypeConversion  OutDataTypeStr=uint8
  Constant8 : Constant  Value=ENUM_VEHICLETYPE_D21
  MVMC_EPSForceSelectD21_Z_enum : Lookup_n-D  BreakpointsForDimension1=AVMC_EPSForceSelectD21_Y_enum  BreakpointsForDimension2=AVMC_EPSForceSelectD21_X_enum  BreakpointsForDimension1DataTypeStr=uint8  BreakpointsForDimension2DataTypeStr=uint8  Table=MVMC_EPSForceSelectD21_Z_enum  TableDataTypeStr=uint8  ExtrapMethod=Clip  InternalRulePriority=Speed  RndMeth=Simplest  InputSameDT=on
      settings: InputPortMap=u0,u1
  MVMC_EPSForceSelect_Z_enum : Lookup_n-D  BreakpointsForDimension1=AVMC_EPSForceSelect_Y_enum  BreakpointsForDimension2=AVMC_EPSForceSelect_X_enum  BreakpointsForDimension1DataTypeStr=uint8  BreakpointsForDimension2DataTypeStr=uint8  Table=MVMC_EPSForceSelect_Z_enum  TableDataTypeStr=uint8  ExtrapMethod=Clip  InternalRulePriority=Speed  RndMeth=Simplest  InputSameDT=on
      settings: InputPortMap=u0,u1
  Relational Operator : RelationalOperator  Operator===  OutDataTypeStr=boolean  RndMeth=Simplest
  Switch : Switch  Criteria=u2 > Threshold
  VVMC_DMSModeCmd_enum : Outport
  wires:
  Switch/1 -> Cast To Single/1
  [VVMC_DMSModeCmd_enum] -> VVMC_DMSModeCmd_enum/1
  VINP_VehicleType_enum/1 -> [VINP_VehicleType_enum]
  VPMM_DrivetrainSelect_enum/1 -> [VPMM_DrivetrainSelect_enum]
  VINP_IVIEPSForceCmd_enum/1 -> [VINP_IVIEPSForceCmd_enum]
  Cast To Single/1 -> [VVMC_DMSModeCmd_enum]  "VVMC_DMSModeCmd_enum"
  MVMC_EPSForceSelect_Z_enum/1 -> Switch/3
  [VINP_IVIEPSForceCmd_enum] -> MVMC_EPSForceSelect_Z_enum/1
  [VINP_VehicleType_enum] -> MVMC_EPSForceSelect_Z_enum/2
  [VPMM_DrivetrainSelect_enum] -> MVMC_EPSForceSelectD21_Z_enum/2
  [VINP_IVIEPSForceCmd_enum] -> MVMC_EPSForceSelectD21_Z_enum/1
  MVMC_EPSForceSelectD21_Z_enum/1 -> Switch/1
  Relational Operator/1 -> Switch/2
  Constant8/1 -> Relational Operator/2
  [VINP_VehicleType_enum] -> Relational Operator/1

== system vmc/VMC/VMC/FeatureSetSpeed ==
  APP_SpdLimit_flg : Inport
  VTQD_SpdCtrlSta_flg : Inport  Port=2
  APP_SpdLimit : Inport  Port=3
  VTQD_SetSpd_kph : Inport  Port=4
  VINP_Distanceunit_flg : Inport  Port=5
  AND : Logic  AllPortsSameDT=off  OutDataTypeStr=boolean
  Cast To Single : DataTypeConversion  OutDataTypeStr=single
  Cast To Single1 : DataTypeConversion  OutDataTypeStr=single
  Constant : Constant  Value=ENUM_SCPCRLSTA_ON
  Constant1 : Constant  Value=ENUM_APPSPDLIMIT_ON
  Constant2 : Constant  Value=ZERO_FLOAT
  Constant3 : Constant  Value=ONE_FLOAT
  Constant4 : Constant  Value=MPH2KPH
  Constant5 : Constant  Value=KVMC_APPSpdLimit_flg_ovrdflg
  Constant6 : Constant  Value=KVMC_APPSpdLimit_flg_ovrdval
  Constant7 : Constant  Value=KVMC_APPSpdLimit_ovrdflg
  Constant8 : Constant  Value=KVMC_APPSpdLimit_ovrdval
  Constant9 : Constant  Value=KVMC_FeatSetSpdKPHRoundSW_flg
  Divide1 : Product  Inputs=**
  Relational Operator : RelationalOperator  Operator=>  OutDataTypeStr=boolean  RndMeth=Simplest
  Round1 : Rounding  Operator=ceil
  Round2 : Rounding  Operator=round
  SpeedDetermination : Stateflow chart  TreatAsAtomicUnit=on
  Switch : Switch  Criteria=u2 ~= 0
  Switch1 : Switch  Criteria=u2 ~= 0
  u2 > 0 (2) : Switch  Criteria=u2 > Threshold
  u2 > 0 (2)1 : Switch  Criteria=u2 > Threshold
  VVMC_FeatSetSpdFinal_raw32 : Outport
  VVMC_FeatSetSpdForCalcu_kph : Outport  Port=2
  wires:
  Relational Operator/1 -> AND/2
  AND/1 -> u2 > 0 (2)/2
  [VVMC_FeatSetSpdFinal_raw32] -> Relational Operator/1
  Constant3/1 -> Relational Operator/2
  VINP_Distanceunit_flg/1 -> [VINP_Distanceunit_flg]
  [VVMC_FeatSetSpdForCalcu_kph] -> VVMC_FeatSetSpdForCalcu_kph/1
  Cast To Single1/1 -> Round2/1, Round1/1
  u2 > 0 (2)1/1 -> [VVMC_FeatSetSpdForCalcu_kph]  "VVMC_FeatSetSpdForCalcu_kph"
  [VINP_Distanceunit_flg] -> AND/1
  Divide1/1 -> u2 > 0 (2)/1
  Constant4/1 -> Divide1/2
  u2 > 0 (2)/1 -> Cast To Single1/1
  [VVMC_FeatSetSpdFinal_raw32] -> u2 > 0 (2)/3, Divide1/1
  [VVMC_FeatSetSpdFinal_raw32] -> VVMC_FeatSetSpdFinal_raw32/1
  VTQD_SetSpd_kph/1 -> [VTQD_SetSpd_kph]
  APP_SpdLimit/1 -> [APP_SpdLimit]
  VTQD_SpdCtrlSta_flg/1 -> [VTQD_SpdCtrlSta_flg]
  APP_SpdLimit_flg/1 -> [APP_SpdLimit_flg]
  [VVMC_APPSpdLimit_kph] -> SpeedDetermination/3(VVMC_APPSpdLimit_kph)
  Cast To Single/1 -> [VVMC_FeatSetSpdFinal_raw32]  "VVMC_FeatSetSpdFinal_raw32"
  Switch/1 -> [VVMC_APPSpdLimit_flg]  "VVMC_APPSpdLimit_flg"
  [VVMC_APPSpdLimit_flg] -> SpeedDetermination/1(VVMC_APPSpdLimit_flg)
  Constant7/1 -> Switch1/2
  [VTQD_SpdCtrlSta_flg] -> SpeedDetermination/2(VTQD_SpdCtrlSta_flg)
  [APP_SpdLimit] -> Switch1/3
  Constant8/1 -> Switch1/1
  Switch1/1 -> [VVMC_APPSpdLimit_kph]  "VVMC_APPSpdLimit_kph"
  Constant/1 -> SpeedDetermination/5(ENUM_SCPCRLSTA_ON)
  SpeedDetermination/1(VVMC_FeatSetSpdFinal_raw32) -> Cast To Single/1
  [APP_SpdLimit_flg] -> Switch/3
  Constant5/1 -> Switch/2
  Constant1/1 -> SpeedDetermination/6(ENUM_APPSPDLIMIT_ON)
  Constant6/1 -> Switch/1
  Constant2/1 -> SpeedDetermination/7(ZERO_FLOAT)
  [VTQD_SetSpd_kph] -> SpeedDetermination/4(VTQD_SetSpd_kph)
  Constant9/1 -> u2 > 0 (2)1/2
  Round1/1 -> u2 > 0 (2)1/3
  Round2/1 -> u2 > 0 (2)1/1

== system vmc/VMC/VMC/IMU ==
  VINP_MemOffsetGyroX_raw16 : Inport
  VINP_MemOffsetGyroY_raw16 : Inport  Port=2
  VINP_MemOffsetGyroZ_raw16 : Inport  Port=3
  VINP_MemOffsetAccX_raw16 : Inport  Port=4
  VINP_MemOffsetAccY_raw16 : Inport  Port=5
  VINP_MemOffsetAccZ_raw16 : Inport  Port=6
  VINP_SensingGyroX_raw16 : Inport  Port=7
  VINP_SensingGyroY_raw16 : Inport  Port=8
  VINP_SensingGyroZ_raw16 : Inport  Port=9
  VINP_SensingAccX_raw16 : Inport  Port=10
  VINP_SensingAccY_raw16 : Inport  Port=11
  VINP_SensingAccZ_raw16 : Inport  Port=12
  task_time_s : Inport  Port=13
  VINP_VehicleType_enum : Inport  Port=14
  Constant : Constant  Value=KVMC_IMUEnaCmd_flg
  Constant1 : Constant  Value=TRUE
  Constant14 : Constant  Value=ENUM_VEHICLETYPE_D31L24
  Equal1 : RelationalOperator  Operator===  OutDataTypeStr=boolean  RndMeth=Simplest
  IMU memorized offset result : Subsystem
  "IMU sensing result " : Subsystem
  Switch1 : Switch  Criteria=u2 > Threshold
  VVMC_IMUEnaCmd_flg : Outport
  VVMC_CalibratedGyroX_Dps : Outport  Port=2
  VVMC_CalibratedGyroY_Dps : Outport  Port=3
  VVMC_CalibratedGyroZ_Dps : Outport  Port=4
  VVMC_CalibratedAccX_G : Outport  Port=5
  VVMC_CalibratedAccY_G : Outport  Port=6
  VVMC_CalibratedAccZ_G : Outport  Port=7
  VVMC_CalibratedAccXAftRA_G : Outport  Port=8
  wires:
  [VVMC_CalibratedAccXAftRA_G] -> VVMC_CalibratedAccXAftRA_G/1
  "IMU sensing result "/7(VVMC_CalibratedAccXAftRA_G) -> [VVMC_CalibratedAccXAftRA_G]
  VINP_VehicleType_enum/1 -> [VINP_VehicleType_enum]
  Constant1/1 -> Switch1/3
  Constant/1 -> Switch1/1
  Equal1/1 -> Switch1/2
  [VINP_VehicleType_enum] -> Equal1/1
  Constant14/1 -> Equal1/2
  [VVMC_CalibratedGyroY_Dps] -> VVMC_CalibratedGyroY_Dps/1
  [VVMC_CalibratedAccY_G] -> VVMC_CalibratedAccY_G/1
  [VVMC_CalibratedGyroZ_Dps] -> VVMC_CalibratedGyroZ_Dps/1
  [VVMC_CalibratedAccZ_G] -> VVMC_CalibratedAccZ_G/1
  [VVMC_CalibratedGyroX_Dps] -> VVMC_CalibratedGyroX_Dps/1
  [VVMC_CalibratedAccX_G] -> VVMC_CalibratedAccX_G/1
  "IMU sensing result "/3(VVMC_CalibratedGyroZ_Dps) -> [VVMC_CalibratedGyroZ_Dps]
  "IMU sensing result "/2(VVMC_CalibratedGyroY_Dps) -> [VVMC_CalibratedGyroY_Dps]
  "IMU sensing result "/6(VVMC_CalibratedAccZ_G) -> [VVMC_CalibratedAccZ_G]
  "IMU sensing result "/5(VVMC_CalibratedAccY_G) -> [VVMC_CalibratedAccY_G]
  "IMU sensing result "/4(VVMC_CalibratedAccX_G) -> [VVMC_CalibratedAccX_G]
  "IMU sensing result "/1(VVMC_CalibratedGyroX_Dps) -> [VVMC_CalibratedGyroX_Dps]
  [task_time_s] -> "IMU sensing result "/13(task_time_s)
  task_time_s/1 -> [task_time_s]
  [VVMC_IMUEnaCmd_flg] -> VVMC_IMUEnaCmd_flg/1
  Switch1/1 -> [VVMC_IMUEnaCmd_flg]  "VVMC_IMUEnaCmd_flg"
  [VINP_SensingGyroY_raw16] -> "IMU sensing result "/2(VINP_SensingGyroY_raw16)
  [VINP_SensingGyroZ_raw16] -> "IMU sensing result "/3(VINP_SensingGyroZ_raw16)
  [VINP_SensingAccX_raw16] -> "IMU sensing result "/4(VINP_SensingAccX_raw16)
  [VINP_SensingAccY_raw16] -> "IMU sensing result "/5(VINP_SensingAccY_raw16)
  [VINP_SensingAccZ_raw16] -> "IMU sensing result "/6(VINP_SensingAccZ_raw16)
  [VINP_SensingGyroX_raw16] -> "IMU sensing result "/1(VINP_SensingGyroX_raw16)
  [VVMC_MemOffsetAccZ_G] -> "IMU sensing result "/12(VVMC_MemOffsetAccZ_G)
  [VVMC_MemOffsetGyroX_Dps] -> "IMU sensing result "/7(VVMC_MemOffsetGyroX_Dps)
  [VVMC_MemOffsetAccY_G] -> "IMU sensing result "/11(VVMC_MemOffsetAccY_G)
  [VVMC_MemOffsetGyroZ_Dps] -> "IMU sensing result "/9(VVMC_MemOffsetGyroZ_Dps)
  [VVMC_MemOffsetAccX_G] -> "IMU sensing result "/10(VVMC_MemOffsetAccX_G)
  [VVMC_MemOffsetGyroY_Dps] -> "IMU sensing result "/8(VVMC_MemOffsetGyroY_Dps)
  IMU memorized offset result/1(VVMC_MemOffsetGyroX_Dps) -> [VVMC_MemOffsetGyroX_Dps]
  IMU memorized offset result/2(VVMC_MemOffsetGyroY_Dps) -> [VVMC_MemOffsetGyroY_Dps]
  IMU memorized offset result/3(VVMC_MemOffsetGyroZ_Dps) -> [VVMC_MemOffsetGyroZ_Dps]
  IMU memorized offset result/4(VVMC_MemOffsetAccX_G) -> [VVMC_MemOffsetAccX_G]
  IMU memorized offset result/5(VVMC_MemOffsetAccY_G) -> [VVMC_MemOffsetAccY_G]
  IMU memorized offset result/6(VVMC_MemOffsetAccZ_G) -> [VVMC_MemOffsetAccZ_G]
  [VINP_MemOffsetAccZ_raw16] -> IMU memorized offset result/6(VINP_MemOffsetAccZ_raw16)
  [VINP_MemOffsetAccY_raw16] -> IMU memorized offset result/5(VINP_MemOffsetAccY_raw16)
  [VINP_MemOffsetAccX_raw16] -> IMU memorized offset result/4(VINP_MemOffsetAccX_raw16)
  [VINP_MemOffsetGyroZ_raw16] -> IMU memorized offset result/3(VINP_MemOffsetGyroZ_raw16)
  [VINP_MemOffsetGyroY_raw16] -> IMU memorized offset result/2(VINP_MemOffsetGyroY_raw16)
  [VINP_MemOffsetGyroX_raw16] -> IMU memorized offset result/1(VINP_MemOffsetGyroX_raw16)
  VINP_SensingAccZ_raw16/1 -> [VINP_SensingAccZ_raw16]
  VINP_SensingAccY_raw16/1 -> [VINP_SensingAccY_raw16]
  VINP_SensingAccX_raw16/1 -> [VINP_SensingAccX_raw16]
  VINP_SensingGyroZ_raw16/1 -> [VINP_SensingGyroZ_raw16]
  VINP_SensingGyroY_raw16/1 -> [VINP_SensingGyroY_raw16]
  VINP_SensingGyroX_raw16/1 -> [VINP_SensingGyroX_raw16]
  VINP_MemOffsetAccZ_raw16/1 -> [VINP_MemOffsetAccZ_raw16]
  VINP_MemOffsetAccY_raw16/1 -> [VINP_MemOffsetAccY_raw16]
  VINP_MemOffsetAccX_raw16/1 -> [VINP_MemOffsetAccX_raw16]
  VINP_MemOffsetGyroZ_raw16/1 -> [VINP_MemOffsetGyroZ_raw16]
  VINP_MemOffsetGyroY_raw16/1 -> [VINP_MemOffsetGyroY_raw16]
  VINP_MemOffsetGyroX_raw16/1 -> [VINP_MemOffsetGyroX_raw16]

== system vmc/VMC/VMC/LFCAOIControl ==
  VINP_APSVRqEPASCtrl_flg : Inport
  VINP_APSRqEPASCtrl_flg : Inport  Port=2
  VINP_ADASStrWhlAngCtrlStatus_flg : Inport  Port=3
  VINP_APSAngleTarget_Deg : Inport  Port=4
  VINP_ADASDesStrWhlAngCtrlCmd_Deg : Inport  Port=5
  VINP_ADASAngCtrlTqWeightGain_pct : Inport  Port=6
  VINP_ADASDrvInputTqBoostAct_flg : Inport  Port=7
  VINP_ADASMaxAngCtrlOutTqLimit_Nm : Inport  Port=8
  VINP_ADASDrvInputTqBoostGain_pct : Inport  Port=9
  VINP_VehicleType_enum : Inport  Port=10
  VDDM_VMCLatCtrlProhibited_flg : Inport  Port=11
  VDDM_VMCEPSErr_flg : Inport  Port=12
  AND{,1..3} (4 alike) : Logic  AllPortsSameDT=off  OutDataTypeStr=boolean
  Cast To Boolean : DataTypeConversion  OutDataTypeStr=boolean
  Cast To Single : DataTypeConversion  OutDataTypeStr=single
  Cast To Single32 : DataTypeConversion  OutDataTypeStr=single
  Constant{1,4,10,12..13} (5 alike) : Constant  Value=ZERO_FLOAT
  Constant11 : Constant  Value=FALSE
  Constant14 : Constant  Value=ENUM_VEHICLETYPE_D31F25
  Constant15 : Constant  Value=ENUM_VEHICLETYPE_D21
  Constant16 : Constant  Value=KVMC_D21AOIAct_flg
  Constant2 : Constant  Value=KVMC_ADASAngCtrlTqWtGnUpperLim_pct
  Constant3 : Constant  Value=KVMC_ADASAngCtrlTqWtGnLowerLim_pct
  Constant5 : Constant  Value=TRUE
  Constant6 : Constant  Value=ENUM_VEHICLETYPE_D31HAWD
  Constant7 : Constant  Value=FALSE
  Constant8 : Constant  Value=ENUM_VEHICLETYPE_D31HRWD
  Constant9 : Constant  Value=FALSE
  Equal{1..4} (4 alike) : RelationalOperator  Operator===  OutDataTypeStr=boolean  RndMeth=Simplest
  NOT : Logic  Operator=NOT  AllPortsSameDT=off  OutDataTypeStr=boolean
  OR : Logic  Operator=OR  Inputs=4  AllPortsSameDT=off  OutDataTypeStr=boolean
  OR1 : Logic  AllPortsSameDT=off  OutDataTypeStr=boolean
  OR2 : Logic  Operator=OR  AllPortsSameDT=off  OutDataTypeStr=boolean
  Saturation Dynamic3 : simulink/Discontinuities/Saturation Dynamic  OutMin=[]  OutMax=[]  OutDataTypeStr=Inherit: Same as second input  OutDataType=fixdt(1, 16)  OutScaling=2^-10  DoSatur=off
  Switch{1..6,9..13} (11 alike) : Switch  Criteria=u2 > Threshold
  VVMC_FDCVMCAPSVRqEPSCtrl_flg : Outport
  VVMC_FDCVMCAPSRqEPSCtrl_flg : Outport  Port=2
  VVMC_FDCVMCAPSAngleTarget_deg : Outport  Port=3
  VVMC_FDCVMCAngCtrlTqWtGn_pct : Outport  Port=4
  VVMC_FDCVMCDrInpTqBstAct_flg : Outport  Port=5
  VVMC_FDCVMCMaxAngCtrlOutTqLim_Nm : Outport  Port=6
  VVMC_FDCVMCDrInpTqBstGn_pct : Outport  Port=7
  wires:
  [VVMC_LFCAOIVehType_flg] -> Switch5/2
  [VVMC_LFCAOIVehType_flg] -> Switch6/2
  [VINP_ADASDrvInputTqBoostGain_pct] -> Switch6/1
  Constant13/1 -> Switch6/3
  [VINP_ADASMaxAngCtrlOutTqLimit_Nm] -> Switch5/1
  Constant12/1 -> Switch5/3
  Constant11/1 -> Switch4/1
  [VDDM_VMCEPSErr_flg] -> Switch4/2
  Switch4/1 -> Switch13/1
  OR2/1 -> Switch13/2
  [VDDM_VMCEPSErr_flg] -> OR2/2
  VDDM_VMCEPSErr_flg/1 -> [VDDM_VMCEPSErr_flg]
  NOT/1 -> OR1/2
  OR/1 -> OR1/1
  [VDDM_VMCLatCtrlProhibited_flg] -> NOT/1
  VDDM_VMCLatCtrlProhibited_flg/1 -> [VDDM_VMCLatCtrlProhibited_flg]
  Switch6/1 -> Cast To Single32/1
  Switch5/1 -> Cast To Single/1
  [VVMC_LFCAOIVehType_flg] -> AND1/2
  AND1/1 -> Cast To Boolean/1
  Saturation Dynamic3/1 -> Switch3/1
  AND2/1 -> Switch3/2
  Constant10/1 -> Switch3/3
  [VINP_ADASStrWhlAngCtrlStatus_flg] -> AND2/1
  [VVMC_LFCAOIVehType_flg] -> AND2/2
  [VVMC_LFCAOIVehType_flg] -> AND/2
  [VINP_ADASStrWhlAngCtrlStatus_flg] -> AND/1
  [VINP_ADASStrWhlAngCtrlStatus_flg] -> Switch2/1
  [VVMC_LFCAOIVehType_flg] -> Switch2/2
  Constant9/1 -> Switch2/3
  Constant7/1 -> Switch1/3
  Switch1/1 -> Switch13/3
  [VVMC_LFCAOIVehType_flg] -> Switch1/2
  OR1/1 -> [VVMC_LFCAOIVehType_flg]  "VVMC_LFCAOIVehType_flg"
  Equal1/1 -> OR/4
  [VINP_VehicleType_enum] -> Equal1/1
  Constant6/1 -> Equal1/2
  [VVMC_FDCVMCAngCtrlTqWtGn_pct] -> VVMC_FDCVMCAngCtrlTqWtGn_pct/1
  [VVMC_FDCVMCDrInpTqBstAct_flg] -> VVMC_FDCVMCDrInpTqBstAct_flg/1
  [VVMC_FDCVMCMaxAngCtrlOutTqLim_Nm] -> VVMC_FDCVMCMaxAngCtrlOutTqLim_Nm/1
  [VVMC_FDCVMCDrInpTqBstGn_pct] -> VVMC_FDCVMCDrInpTqBstGn_pct/1
  [VVMC_FDCVMCAPSAngleTarget_deg] -> VVMC_FDCVMCAPSAngleTarget_deg/1
  [VVMC_FDCVMCAPSRqEPSCtrl_flg] -> VVMC_FDCVMCAPSRqEPSCtrl_flg/1
  [VVMC_FDCVMCAPSVRqEPSCtrl_flg] -> VVMC_FDCVMCAPSVRqEPSCtrl_flg/1
  VINP_VehicleType_enum/1 -> [VINP_VehicleType_enum]
  VINP_ADASDrvInputTqBoostGain_pct/1 -> [VINP_ADASDrvInputTqBoostGain_pct]
  VINP_ADASStrWhlAngCtrlStatus_flg/1 -> [VINP_ADASStrWhlAngCtrlStatus_flg]
  VINP_APSAngleTarget_Deg/1 -> [VINP_APSAngleTarget_Deg]
  VINP_ADASDesStrWhlAngCtrlCmd_Deg/1 -> [VINP_ADASDesStrWhlAngCtrlCmd_Deg]
  VINP_ADASAngCtrlTqWeightGain_pct/1 -> [VINP_ADASAngCtrlTqWeightGain_pct]
  VINP_ADASDrvInputTqBoostAct_flg/1 -> [VINP_ADASDrvInputTqBoostAct_flg]
  VINP_ADASMaxAngCtrlOutTqLimit_Nm/1 -> [VINP_ADASMaxAngCtrlOutTqLimit_Nm]
  VINP_APSVRqEPASCtrl_flg/1 -> [VINP_APSVRqEPASCtrl_flg]
  VINP_APSRqEPASCtrl_flg/1 -> [VINP_APSRqEPASCtrl_flg]
  Constant5/1 -> Switch1/1
  Constant8/1 -> Equal3/2
  [VINP_ADASDrvInputTqBoostAct_flg] -> AND1/1
  Switch3/1 -> Switch12/3
  [VINP_APSRqEPASCtrl_flg] -> Switch9/2
  Cast To Boolean/1 -> [VVMC_FDCVMCDrInpTqBstAct_flg]  "VVMC_FDCVMCDrInpTqBstAct_flg"
  Constant3/1 -> Saturation Dynamic3/3
  [VINP_ADASAngCtrlTqWeightGain_pct] -> Saturation Dynamic3/2
  [VINP_APSVRqEPASCtrl_flg] -> OR2/1, Switch4/3
  Constant2/1 -> Saturation Dynamic3/1
  Constant1/1 -> Switch12/1
  Switch13/1 -> [VVMC_FDCVMCAPSVRqEPSCtrl_flg]  "VVMC_FDCVMCAPSVRqEPSCtrl_flg"
  [VINP_VehicleType_enum] -> Equal3/1
  [VINP_APSRqEPASCtrl_flg] -> Switch10/1
  Equal3/1 -> OR/3
  Constant4/1 -> Switch11/3
  [VINP_ADASDesStrWhlAngCtrlCmd_Deg] -> Switch11/1
  Switch10/1 -> [VVMC_FDCVMCAPSRqEPSCtrl_flg]  "VVMC_FDCVMCAPSRqEPSCtrl_flg"
  [VINP_APSRqEPASCtrl_flg] -> Switch12/2
  Cast To Single32/1 -> [VVMC_FDCVMCDrInpTqBstGn_pct]  "VVMC_FDCVMCDrInpTqBstGn_pct"
  Switch2/1 -> Switch10/3
  [VINP_APSRqEPASCtrl_flg] -> Switch10/2
  Cast To Single/1 -> [VVMC_FDCVMCMaxAngCtrlOutTqLim_Nm]  "VVMC_FDCVMCMaxAngCtrlOutTqLim_Nm"
  Switch9/1 -> [VVMC_FDCVMCAPSAngleTarget_deg]  "VVMC_FDCVMCAPSAngleTarget_deg"
  Switch12/1 -> [VVMC_FDCVMCAngCtrlTqWtGn_pct]  "VVMC_FDCVMCAngCtrlTqWtGn_pct"
  AND/1 -> Switch11/2
  Switch11/1 -> Switch9/3
  [VINP_APSAngleTarget_Deg] -> Switch9/1
  [VINP_VehicleType_enum] -> Equal2/1
  Constant14/1 -> Equal2/2
  Equal2/1 -> OR/2
  Constant15/1 -> Equal4/2
  [VINP_VehicleType_enum] -> Equal4/1
  Equal4/1 -> AND3/1
  Constant16/1 -> AND3/2
  AND3/1 -> OR/1
